simulink model "wheelspeedsim"  (R2015b)
settings: Solver=ode1  StartTime=0.0  StopTime=Inf  FixedStep=0.001  RelTol=1e-3
PostLoadFcn:
  | , if any(exist('dsrtsu_mdlpostloadfcn', 'file') == [2, 3, 6]), try dsrtsu_mdlpostloadfcn('Execute', bdroot); catch fprintf('Error in PostLoadFcn (dsrtsu_mdlpostloadfcn) for model "%s":\n %s\n', bdroot, lasterr); end, end,
values from neighbouring files (symbols this model uses):
  FL_Speed = 0.0    (= 0)    [wheelspeedsim_init.m]
  FR_Speed = 0.0    (= 0)    [wheelspeedsim_init.m]
  RL_Speed = 0.0    (= 0)    [wheelspeedsim_init.m]
  RR_Speed = 0.0    (= 0)    [wheelspeedsim_init.m]
undefined symbols (not defined in the file or in its folder): h, km, m, s
libraries: rti1401lib_dio_type4 x6, aerolibconvert2 x5, dspswit3 x1
settings Model: DSRTSU_INTERNAL_RTI_VER=460  DSRTSU_INTERNAL_RTI_TYPE=rti1401  DSRTSU_INTERNAL_RTIFPGA=50  Creator=luis  LastModifiedBy=luis
settings OptimizationCC: BlockReduction=off  OptimizeBlockIOStorage=off  BufferReuse=off  GlobalBufferReuse=off  ExpressionFolding=off  LocalBlockOutputs=off
settings HardwareCC: ProdEndianess=BigEndian  ProdWordSize=32  ProdHWDeviceType=Generic->Custom  TargetIntDivRoundTo=Zero  TargetEndianess=BigEndian  TargetHWDeviceType=Generic->Custom
settings RTWCC: SystemTargetFile=rti1401.tlc  MakeCommand=make_rti  TemplateMakefile=rti1401.tmf  Description=dSPACE DS1401 Hardware Platform
settings STFCustomTargetCC: ParMdlRefBuildCompliant=on  ConcurrentExecutionCompliant=off  GeneratePreprocessorConditionals=Use local settings  CPPClassGenCompliant=off  SystemTargetFile=rti1401.tlc
settings GRTTargetCC: CompOptLevelCompliant=off  ConcurrentExecutionCompliant=off  CombineOutputUpdateFcns=off  MatFileLogging=off  CPPClassGenCompliant=off  GRTInterface=on  UseToolchainInfoCompliant=off  ExtModeMexFile=noextcomm

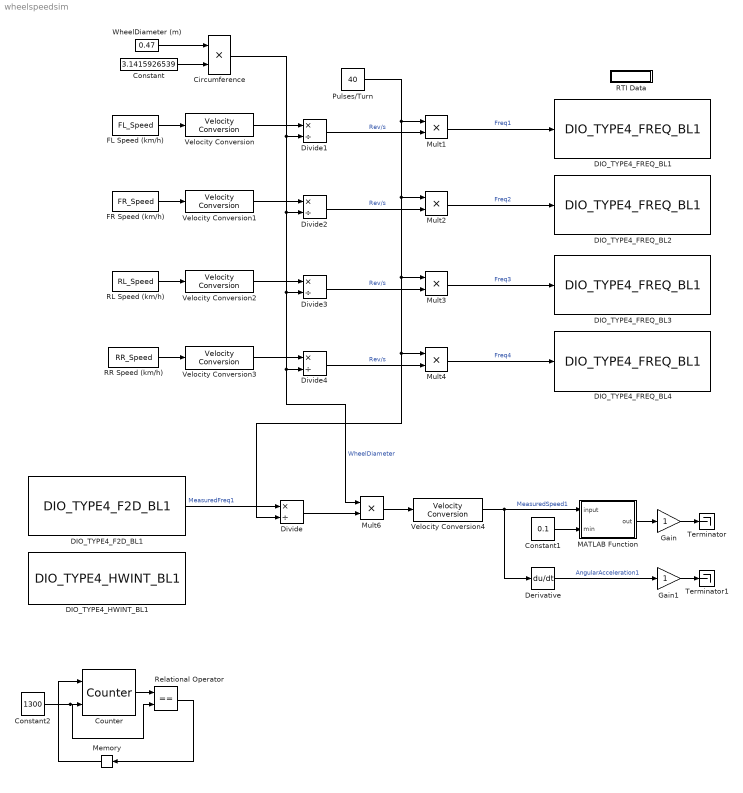
== system wheelspeedsim ==
  Circumference : Product
  Constant : Constant  Value=3.1415926539
  Constant1 : Constant  Value=0.1
  Constant2 : Constant  Value=1300
  Counter : dspswit3/Counter  Direction=Up  CountEvent=Free running  CounterSize=Specify via input port  MaxCount=1300  InitialCount=0  Output=Count  HitValue=1300  ResetInput=on  SamplesPerFrame=1  Ts=-1  CntDtype=double  HitDtype=Logical
  DIO_TYPE4_F2D_BL1 : rti1401lib_dio_type4/DIO_TYPE4_F2D_BL1  DSProperties=struct('RTI',struct('Version',uint32(1),'BlockType',struct('isSLSource',uint8(1),'isSLSink',uint8(0),'isHWSource',uint8(1),'isHWSink',uint8(0),'isSetup',uint8(0),'isInline',uint8(1),'isNonInline',uint8(0),'isInterrupt',uint8(0),'isChannelwise',uint8(1)),'IOBoardType',{{'DS1401','STD','DIOT4'}},'UnitType','PWM','Identifier','F2D','DialogType','ML','BlockSet','NONE','SlaveProcessor','NONE'))  RTIBlockInterface=struct('OutputPortsWidth',int32(1),'OutputPortsActive',1,'OutputPortsName',{{'Frequency'}},'BlockDisplay',{{['DIO TP4 F2D\nModule: 1\nPort: 1\nChannel: 1'],'center'}},'IconTransparency','on','InitLevel',3,'DialogFcn','rti1401stddiot4f2dgui','BlockName',struct('Token',{{'DIO_TYPE4_F2D_BL1'}}))  RTIBlockParameters=struct('ModuleNo',{{1,'ON',[1 16]}},'PortNo',{{1,'OFF',[1 2]}},'ChannelNo',{{1,'ON',[1 16]}},'FrequencyRange',{{8,'OFF',[1 16]}},'TLCFileName',{{'rti1401dio_t4_f2d','OFF',[]}},'EnableInterrupt',{{1,'OFF',[0 1]}},'TriggerEdgeType',{{2,'OFF',[1 3]}})  RTISFcnParameters=struct('ModuleNo','int32','PortNo','int16','ChannelNo','int16','FrequencyRange','int16','TLCFileName','char','EnableInterrupt','int16','TriggerEdgeType','int32')  RTIBlockParaDefault=struct('ModuleNo',1,'PortNo',1,'ChannelNo',1,'FrequencyRange',1,'TLCFileName','rti1401dio_t4_f2d','EnableInterrupt',0,'TriggerEdgeType',1)
  DIO_TYPE4_FREQ_BL1 : rti1401lib_dio_type4/DIO_TYPE4_FREQ_BL1  DSProperties=struct('RTI',struct('Version',uint32(1),'BlockType',struct('isSLSource',uint8(0),'isSLSink',uint8(1),'isHWSource',uint8(0),'isHWSink',uint8(1),'isSetup',uint8(0),'isInline',uint8(1),'isNonInline',uint8(0),'isInterrupt',uint8(0),'isChannelwise',uint8(1)),'IOBoardType',{{'DS1401','STD','DIOT4'}},'UnitType','PWM','Identifier','FREQ','DialogType','ML','BlockSet','NONE','SlaveProcessor','NONE'))  RTIBlockInterface=struct('InputPortsWidth',int32(1),'InputPortsActive',1,'InputPortsName',{{'Frequency'}},'BlockDisplay',{{['DIO TP4 FREQ OUT\nModule: 1\nPort: 1\nChannel: 1'],'center'}},'IconTransparency','on','InitLevel',3,'DialogFcn','rti1401stddiot4freqgui','BlockName',struct('Token',{{'DIO_TYPE4_FREQ_BL1'}}))  RTIBlockParameters=struct('ModuleNo',{{1,'ON',[1 16]}},'PortNo',{{1,'OFF',[1 2]}},'ChannelNo',{{1,'ON',[1 16]}},'SupplyRailsCh',{{[1 1],'OFF',[0 1 0 1]}},'FrequencyRange',{{8,'OFF',[1 16]}},'FrequencyInit',{{'0','OFF',[]}},'OutputModeOnZero',{{1,'OFF',[1 3]}},'TerminationMode',{{0,'OFF',[0 1]}},'OutputTermValidate',{{0,'OFF',[0 1]}},'OutputTermBuildCheck',{{0,'OFF',[]}},'FrequencyTerm',{{'0','OFF',[]}},'TLCFileName',{{'rti1401dio_t4_freq','OFF',[]}},'EnableInterrupt',{{0,'OFF',[0 1]}},'TriggerEdgeType',{{1,'OFF',[1 3]}})  RTISFcnParameters=struct('ModuleNo','int32','PortNo','int16','ChannelNo','int16','SupplyRailsCh','int16','FrequencyRange','int16','FrequencyInit','double','OutputModeOnZero','int16','TerminationMode','int16','OutputTermValidate','int16','FrequencyTerm','double','TLCFileName','char','EnableInterrupt','int16','TriggerEdgeType','int32')  RTIBlockParaDefault=struct('ModuleNo',1,'PortNo',1,'ChannelNo',1,'SupplyRailsCh',[1 1],'FrequencyRange',1,'FrequencyInit',0,'OutputModeOnZero',1,'TerminationMode',0,'OutputTermValidate',0,'OutputTermBuildCheck',0,'FrequencyTerm',0,'TLCFileName','rti1401dio_t4_freq','EnableInterrupt',0,'TriggerEdgeType',1)
  DIO_TYPE4_FREQ_BL2 : rti1401lib_dio_type4/DIO_TYPE4_FREQ_BL1  DSProperties=struct('RTI',struct('Version',uint32(1),'BlockType',struct('isSLSource',uint8(0),'isSLSink',uint8(1),'isHWSource',uint8(0),'isHWSink',uint8(1),'isSetup',uint8(0),'isInline',uint8(1),'isNonInline',uint8(0),'isInterrupt',uint8(0),'isChannelwise',uint8(1)),'IOBoardType',{{'DS1401','STD','DIOT4'}},'UnitType','PWM','Identifier','FREQ','DialogType','ML','BlockSet','NONE','SlaveProcessor','NONE'))  RTIBlockInterface=struct('InputPortsWidth',int32(1),'InputPortsActive',1,'InputPortsName',{{'Frequency'}},'BlockDisplay',{{['DIO TP4 FREQ OUT\nModule: 1\nPort: 1\nChannel: 2'],'center'}},'IconTransparency','on','InitLevel',3,'DialogFcn','rti1401stddiot4freqgui','BlockName',struct('Token',{{'DIO_TYPE4_FREQ_BL1'}}))  RTIBlockParameters=struct('ModuleNo',{{1,'ON',[1 16]}},'PortNo',{{1,'OFF',[1 2]}},'ChannelNo',{{2,'ON',[1 16]}},'SupplyRailsCh',{{[1 1],'OFF',[0 1 0 1]}},'FrequencyRange',{{8,'OFF',[1 16]}},'FrequencyInit',{{'0','OFF',[]}},'OutputModeOnZero',{{1,'OFF',[1 3]}},'TerminationMode',{{0,'OFF',[0 1]}},'OutputTermValidate',{{0,'OFF',[0 1]}},'OutputTermBuildCheck',{{0,'OFF',[]}},'FrequencyTerm',{{'0','OFF',[]}},'TLCFileName',{{'rti1401dio_t4_freq','OFF',[]}},'EnableInterrupt',{{0,'OFF',[0 1]}},'TriggerEdgeType',{{1,'OFF',[1 3]}})  RTISFcnParameters=struct('ModuleNo','int32','PortNo','int16','ChannelNo','int16','SupplyRailsCh','int16','FrequencyRange','int16','FrequencyInit','double','OutputModeOnZero','int16','TerminationMode','int16','OutputTermValidate','int16','FrequencyTerm','double','TLCFileName','char','EnableInterrupt','int16','TriggerEdgeType','int32')  RTIBlockParaDefault=struct('ModuleNo',1,'PortNo',1,'ChannelNo',1,'SupplyRailsCh',[1 1],'FrequencyRange',1,'FrequencyInit',0,'OutputModeOnZero',1,'TerminationMode',0,'OutputTermValidate',0,'OutputTermBuildCheck',0,'FrequencyTerm',0,'TLCFileName','rti1401dio_t4_freq','EnableInterrupt',0,'TriggerEdgeType',1)
  DIO_TYPE4_FREQ_BL3 : rti1401lib_dio_type4/DIO_TYPE4_FREQ_BL1  DSProperties=struct('RTI',struct('Version',uint32(1),'BlockType',struct('isSLSource',uint8(0),'isSLSink',uint8(1),'isHWSource',uint8(0),'isHWSink',uint8(1),'isSetup',uint8(0),'isInline',uint8(1),'isNonInline',uint8(0),'isInterrupt',uint8(0),'isChannelwise',uint8(1)),'IOBoardType',{{'DS1401','STD','DIOT4'}},'UnitType','PWM','Identifier','FREQ','DialogType','ML','BlockSet','NONE','SlaveProcessor','NONE'))  RTIBlockInterface=struct('InputPortsWidth',int32(1),'InputPortsActive',1,'InputPortsName',{{'Frequency'}},'BlockDisplay',{{['DIO TP4 FREQ OUT\nModule: 1\nPort: 1\nChannel: 3'],'center'}},'IconTransparency','on','InitLevel',3,'DialogFcn','rti1401stddiot4freqgui','BlockName',struct('Token',{{'DIO_TYPE4_FREQ_BL1'}}))  RTIBlockParameters=struct('ModuleNo',{{1,'ON',[1 16]}},'PortNo',{{1,'OFF',[1 2]}},'ChannelNo',{{3,'ON',[1 16]}},'SupplyRailsCh',{{[1 1],'OFF',[0 1 0 1]}},'FrequencyRange',{{8,'OFF',[1 16]}},'FrequencyInit',{{'0','OFF',[]}},'OutputModeOnZero',{{1,'OFF',[1 3]}},'TerminationMode',{{0,'OFF',[0 1]}},'OutputTermValidate',{{0,'OFF',[0 1]}},'OutputTermBuildCheck',{{0,'OFF',[]}},'FrequencyTerm',{{'0','OFF',[]}},'TLCFileName',{{'rti1401dio_t4_freq','OFF',[]}},'EnableInterrupt',{{0,'OFF',[0 1]}},'TriggerEdgeType',{{1,'OFF',[1 3]}})  RTISFcnParameters=struct('ModuleNo','int32','PortNo','int16','ChannelNo','int16','SupplyRailsCh','int16','FrequencyRange','int16','FrequencyInit','double','OutputModeOnZero','int16','TerminationMode','int16','OutputTermValidate','int16','FrequencyTerm','double','TLCFileName','char','EnableInterrupt','int16','TriggerEdgeType','int32')  RTIBlockParaDefault=struct('ModuleNo',1,'PortNo',1,'ChannelNo',1,'SupplyRailsCh',[1 1],'FrequencyRange',1,'FrequencyInit',0,'OutputModeOnZero',1,'TerminationMode',0,'OutputTermValidate',0,'OutputTermBuildCheck',0,'FrequencyTerm',0,'TLCFileName','rti1401dio_t4_freq','EnableInterrupt',0,'TriggerEdgeType',1)
  DIO_TYPE4_FREQ_BL4 : rti1401lib_dio_type4/DIO_TYPE4_FREQ_BL1  DSProperties=struct('RTI',struct('Version',uint32(1),'BlockType',struct('isSLSource',uint8(0),'isSLSink',uint8(1),'isHWSource',uint8(0),'isHWSink',uint8(1),'isSetup',uint8(0),'isInline',uint8(1),'isNonInline',uint8(0),'isInterrupt',uint8(0),'isChannelwise',uint8(1)),'IOBoardType',{{'DS1401','STD','DIOT4'}},'UnitType','PWM','Identifier','FREQ','DialogType','ML','BlockSet','NONE','SlaveProcessor','NONE'))  RTIBlockInterface=struct('InputPortsWidth',int32(1),'InputPortsActive',1,'InputPortsName',{{'Frequency'}},'BlockDisplay',{{['DIO TP4 FREQ OUT\nModule: 1\nPort: 1\nChannel: 4'],'center'}},'IconTransparency','on','InitLevel',3,'DialogFcn','rti1401stddiot4freqgui','BlockName',struct('Token',{{'DIO_TYPE4_FREQ_BL1'}}))  RTIBlockParameters=struct('ModuleNo',{{1,'ON',[1 16]}},'PortNo',{{1,'OFF',[1 2]}},'ChannelNo',{{4,'ON',[1 16]}},'SupplyRailsCh',{{[1 1],'OFF',[0 1 0 1]}},'FrequencyRange',{{8,'OFF',[1 16]}},'FrequencyInit',{{'0','OFF',[]}},'OutputModeOnZero',{{1,'OFF',[1 3]}},'TerminationMode',{{0,'OFF',[0 1]}},'OutputTermValidate',{{0,'OFF',[0 1]}},'OutputTermBuildCheck',{{0,'OFF',[]}},'FrequencyTerm',{{'0','OFF',[]}},'TLCFileName',{{'rti1401dio_t4_freq','OFF',[]}},'EnableInterrupt',{{0,'OFF',[0 1]}},'TriggerEdgeType',{{1,'OFF',[1 3]}})  RTISFcnParameters=struct('ModuleNo','int32','PortNo','int16','ChannelNo','int16','SupplyRailsCh','int16','FrequencyRange','int16','FrequencyInit','double','OutputModeOnZero','int16','TerminationMode','int16','OutputTermValidate','int16','FrequencyTerm','double','TLCFileName','char','EnableInterrupt','int16','TriggerEdgeType','int32')  RTIBlockParaDefault=struct('ModuleNo',1,'PortNo',1,'ChannelNo',1,'SupplyRailsCh',[1 1],'FrequencyRange',1,'FrequencyInit',0,'OutputModeOnZero',1,'TerminationMode',0,'OutputTermValidate',0,'OutputTermBuildCheck',0,'FrequencyTerm',0,'TLCFileName','rti1401dio_t4_freq','EnableInterrupt',0,'TriggerEdgeType',1)
  DIO_TYPE4_HWINT_BL1 : rti1401lib_dio_type4/DIO_TYPE4_HWINT_BL1  DSProperties=struct('RTI',struct('Version',uint32(1),'BlockType',struct('isSLSource',uint8(1),'isSLSink',uint8(0),'isHWSource',uint8(0),'isHWSink',uint8(0),'isSetup',uint8(0),'isInline',uint8(1),'isNonInline',uint8(0),'isInterrupt',uint8(1),'isChannelwise',uint8(0)),'IOBoardType',{{'DS1401','STD','DIOT4'}},'UnitType','DSTASKTOOL','Identifier','HWINT','DialogType','ML','BlockSet','NONE','SlaveProcessor','NONE'))  RTIBlockInterface=struct('OutputPortsActive',1,'OutputPortsWidth',int32(1),'OutputPortsName',{{'Interrupt'}},'FunctionCall',uint32(0),'DialogFcn','rti1401stddiot4hwintgui','InitLevel',3,'BlockDisplay',{{['DIO TP4 HW INT\nModule: 1\nPort: 1\nInput channel: 1'],'center'}},'IconTransparency','on','BlockName',struct('Token',{{'DIO_TYPE4_HWINT_BL1'}}))  RTIBlockParameters=struct('ModuleNo',{{1,'OFF',[1 16]}},'PortNo',{{1,'ON',[1 2]}},'ChannelNo',{{1,'ON',[1 16]}},'ChannelDirection',{{1,'ON',[1 2]}})  RTISFcnParameters=struct('ModuleNo','int32','PortNo','int32','ChannelNo','int32','ChannelDirection','int32')  RTIBlockParaDefault=struct('ModuleNo',1,'PortNo',1,'ChannelNo',1,'ChannelDirection',1)
  Derivative : Derivative  CoefficientInTFapproximation=1
  Divide{,1..4} (5 alike) : Product  Inputs=*/
  FL Speed (km/h) : Constant  Value=FL_Speed
  FR Speed (km/h) : Constant  Value=FR_Speed
  Gain : Gain
  Gain1 : Gain
  MATLAB Function : MATLAB Function  TreatAsAtomicUnit=on
  Memory : Memory
  Mult{1..4,6} (5 alike) : Product
  Pulses/Turn : Constant  Value=40
  RL Speed (km/h) : Constant  Value=RL_Speed
  RR Speed (km/h) : Constant  Value=RR_Speed
  RTI Data : Subsystem  Tag=struct('RTIDataServer',struct('RTIDataServerVs','2','RTIModelDescription','struct(''main'',''wheelspeedsim'',''sub'','''',''isMp'',0)'))  LoadFcn="if exist('rtidc'), try,  rtidc('DataHostBlockClbLoad', gcbh); catch, disp(['Warning: ''LoadFcn'' for RTI Data block failed: ' lasterr]); end, end,"  mask(RTI_DATA_HOST){}
      mask help:
      | RTI Data Block.
      | This block is used by RTI to store internal model-dependent data.
      | Please keep this block on the root level of the model. Deleting this block will result in data loss.
      |
      | NEVER DELETE OR COPY THIS BLOCK!
      settings: CopyFcn="if exist('rtidc'), try,  rtidc('DataHostBlockClbCopy', gcbh); catch, disp(['Warning: ''CopyFcn'' for RTI Data block failed: ' lasterr]); end, end,"  DeleteFcn="if exist('rtidc'), try,  rtidc('DataHostBlockClbDelete', gcbh); catch, disp(['Warning: ''DeleteFcn'' for RTI Data block failed: ' lasterr]); end, end,"  ModelCloseFcn="if exist('rtidc'), try,  rtidc('DataHostBlockClbModelClose', gcbh); catch, disp(['Warning: ''ModelCloseFcn'' for RTI Data block failed: ' lasterr]); end, end,"  PreSaveFcn="if exist('rtidc'), try,  rtidc('DataHostBlockClbPreSave', gcbh); catch, disp(['Warning: ''PreSaveFcn'' for RTI Data block failed: ' lasterr]); end, end,"  PostSaveFcn="if exist('rtidc'), try,  rtidc('DataHostBlockClbPostSave', gcbh); catch, disp(['Warning: ''PostSaveFcn'' for RTI Data block failed: ' lasterr]); end, end,"  NameChangeFcn="if exist('rtidc'), try,  rtidc('DataHostBlockClbNameChange', gcbh); catch, disp(['Warning: ''NameChangeFcn'' for RTI Data block failed: ' lasterr]); end, end,"
      mask Help:
      | RTI Data Block.
      | This block is used by RTI to store internal model-dependent data.
      | Please keep this block on the root level of the model. Deleting this block will result in data loss.
      | 
      | NEVER DELETE OR COPY THIS BLOCK!
      mask Display:
      | text(0.5, 0.5, 'RTI Data', 'HorizontalAlignment', 'center');
      | plot([1 0]);
  Relational Operator : RelationalOperator  Operator===  OutDataTypeStr=boolean
  Terminator : Terminator
  Terminator1 : Terminator
  Velocity Conversion{,1..3} (4 alike) : aerolibconvert2/Velocity Conversion  IU=km/h  OU=m/s
  Velocity Conversion4 : aerolibconvert2/Velocity Conversion  IU=m/s  OU=km/h
  WheelDiameter (m) : Constant  Value=0.47
  wires:
  FL Speed (km/h)/1 -> Velocity Conversion/1
  WheelDiameter (m)/1 -> Circumference/1
  Constant/1 -> Circumference/2
  Circumference/1 -> Divide4/2, Mult6/1, Divide3/2, Divide2/2, Divide1/2  "WheelDiameter"
  Velocity Conversion/1 -> Divide1/1
  Divide1/1 -> Mult1/2  "Rev/s"
  Pulses/Turn/1 -> Mult1/1, Divide/2, Mult4/1, Mult3/1, Mult2/1
  Mult1/1 -> DIO_TYPE4_FREQ_BL1/1  "Freq1"
  Velocity Conversion1/1 -> Divide2/1
  Divide2/1 -> Mult2/2  "Rev/s"
  Mult2/1 -> DIO_TYPE4_FREQ_BL2/1  "Freq2"
  FR Speed (km/h)/1 -> Velocity Conversion1/1
  Velocity Conversion2/1 -> Divide3/1
  Divide3/1 -> Mult3/2  "Rev/s"
  Mult3/1 -> DIO_TYPE4_FREQ_BL3/1  "Freq3"
  RL Speed (km/h)/1 -> Velocity Conversion2/1
  Velocity Conversion3/1 -> Divide4/1
  Divide4/1 -> Mult4/2  "Rev/s"
  Mult4/1 -> DIO_TYPE4_FREQ_BL4/1  "Freq4"
  RR Speed (km/h)/1 -> Velocity Conversion3/1
  DIO_TYPE4_F2D_BL1/1 -> Divide/1  "MeasuredFreq1"
  Divide/1 -> Mult6/2
  Mult6/1 -> Velocity Conversion4/1
  Velocity Conversion4/1 -> MATLAB Function/1(input), Derivative/1  "MeasuredSpeed1"
  Gain/1 -> Terminator/1
  Counter/1 -> Relational Operator/1
  Constant2/1 -> Relational Operator/2, Counter/2
  Relational Operator/1 -> Memory/1
  Memory/1 -> Counter/1
  Derivative/1 -> Gain1/1  "AngularAcceleration1"
  Gain1/1 -> Terminator1/1
  MATLAB Function/1(out) -> Gain/1
  Constant1/1 -> MATLAB Function/2(min)

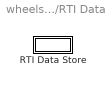
== system wheelspeedsim/RTI Data ==
  RTI Data Store : Subsystem  Tag="struct('private',struct('version',struct('dsVer',uint32(2),'dsVerCreation',uint32(2),'RTI',struct('ver','7.4','type','RTI1401')),'access',struct('type','Model','isPerm',1,'created',['24-Mar-2017 13:01:57'],'modified',['27-Mar-2017 21:50:33'],'location','')),'public',struct('main',struct('data',[]),'sub',struct('name',{{'wheelspeedsim'}},'data',{{struct('TH',struct('thTaskInfo',struct('taskType',{'TIMER','HWINT','TMRINT','SWINT','GLINT'},'tasksNumOf',{1,0,0,0,0},'srcIds',{{'TIMERA'},{},{},{},{}},'taskNames',{{['Timer Task 1']},{},{},{},{}})),'th_tc',struct('dataType','TASK','taskGroupId','','taskGroupList',{{}},'taskSchedulingPolicy','FCFS','taskType','TIMER','blkh',-1,'srcId','TIMERA','srcSgnName',['Timer A interrupt'],'srcCpuName','','taskName',['Timer Task 1  [0.001] s'],'taskNameDisplayExt','','smplTime',0.001,'smplTimeOffs',0,'hasFixedPriority',0,'priority',1,'hasFixedOvc',0,'ovcType',1,'ovcMax',1),'tc_th',struct('dataType','TASK','taskGroupId','','taskGroupList',{{}},'taskSchedulingPolicy','FCFS','taskType','TIMER','blkh',-1,'srcId','TIMERA','srcSgnName',['Timer A interrupt'],'srcCpuName','','taskName',['Timer Task 1  [0.001] s'],'taskNameDisplayExt','','smplTime',0.001,'smplTimeOffs',0,'hasFixedPriority',0,'priority',1,'hasFixedOvc',0,'ovcType',1,'ovcMax',1))}})))"  mask(RTI_DATA_STORE){}
      mask help:
      | RTI Data Store Block. This block is used by RTI to store internal model dependent data. Deleting this block will result in data loss.
      |
      | NEVER DELETE, COPY, OR MODIFY THIS BLOCK!
      mask Help:
      | RTI Data Store Block. This block is used by RTI to store internal model dependent data. Deleting this block will result in data loss.
      | 
      | NEVER DELETE, COPY, OR MODIFY THIS BLOCK!
      mask Display: text(0.5, 0.5, ' ', 'HorizontalAlignment', 'center');

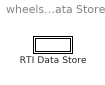
== system wheelspeedsim/RTI Data/RTI Data Store ==
  RTI Data Store : Subsystem  mask(RTI_DATA_STORE){}
      mask help:
      | RTI Data Store Block. This block is used by RTI to store internal model dependent data. Deleting this block will result in data loss.
      |
      | NEVER DELETE, COPY, OR MODIFY THIS BLOCK!
      mask Help:
      | RTI Data Store Block. This block is used by RTI to store internal model dependent data. Deleting this block will result in data loss.
      | 
      | NEVER DELETE, COPY, OR MODIFY THIS BLOCK!
      mask Display: text(0.5, 0.5, ' ', 'HorizontalAlignment', 'center');

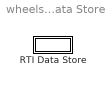
== system wheelspeedsim/RTI Data/RTI Data Store/RTI Data Store ==
  RTI Data Store : Subsystem  mask(RTI_DATA_STORE){}
      mask help:
      | RTI Data Store Block. This block is used by RTI to store internal model dependent data. Deleting this block will result in data loss.
      |
      | NEVER DELETE, COPY, OR MODIFY THIS BLOCK!
      mask Help:
      | RTI Data Store Block. This block is used by RTI to store internal model dependent data. Deleting this block will result in data loss.
      | 
      | NEVER DELETE, COPY, OR MODIFY THIS BLOCK!
      mask Display: text(0.5, 0.5, ' ', 'HorizontalAlignment', 'center');

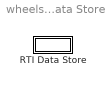
== system wheelspeedsim/RTI Data/RTI Data Store/RTI Data Store/RTI Data Store ==
  RTI Data Store : Subsystem  mask(RTI_DATA_STORE){}
      mask help:
      | RTI Data Store Block. This block is used by RTI to store internal model dependent data. Deleting this block will result in data loss.
      |
      | NEVER DELETE, COPY, OR MODIFY THIS BLOCK!
      mask Help:
      | RTI Data Store Block. This block is used by RTI to store internal model dependent data. Deleting this block will result in data loss.
      | 
      | NEVER DELETE, COPY, OR MODIFY THIS BLOCK!
      mask Display: text(0.5, 0.5, ' ', 'HorizontalAlignment', 'center');

== system wheelspeedsim/RTI Data/RTI Data Store/RTI Data Store/RTI Data Store/RTI Data Store ==

== matlab function wheelspeedsim/MATLAB Function ==
  data: input input; out output; min input
function out = fcn(input, min)
%#codegen
out = input;
if input < min
    out = 0.0;
end
